simulink model "DeratingControl"  (R2021b)
settings: Solver=VariableStepAuto  StartTime=0.0  StopTime=2  FixedStep=Ts  RelTol=1e-3
model workspace (MAT data in the model file):
  df = Simulink.Parameter
  df.Value = 0.9
  df.DataType = 'auto'
  df.Complexity = 'real'
  df.Dimensions = [1 1]
undefined symbols (not defined in the file): const_facInvTempDera, const_facMotTempDera, const_facPwrDera, const_stDera, const_tiTaskFast, const_tqBattDeraGenLim, const_tqBattDeraMotLim, const_tqDeraGen, const_tqDeraMot, const_tqEmMaxNp1, const_tqInvTempDeraMax, const_tqInvTempDeraMin, const_tqMotTempDeraMax, const_tqMotTempDeraMin, const_tqSpLim, const_tqSpLimMax, const_tqSpLimMin, const_tqTqReq
libraries: simulink x3
settings Model: PacingRate=0.350000  Creator=win  LastModifiedBy=win

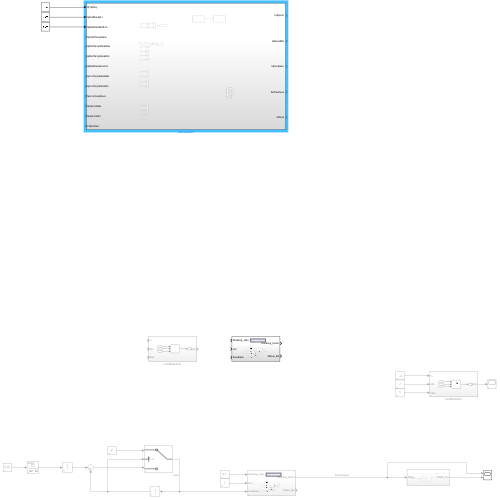
[thumbnail: Simulink's stored preview of the top-level diagram]
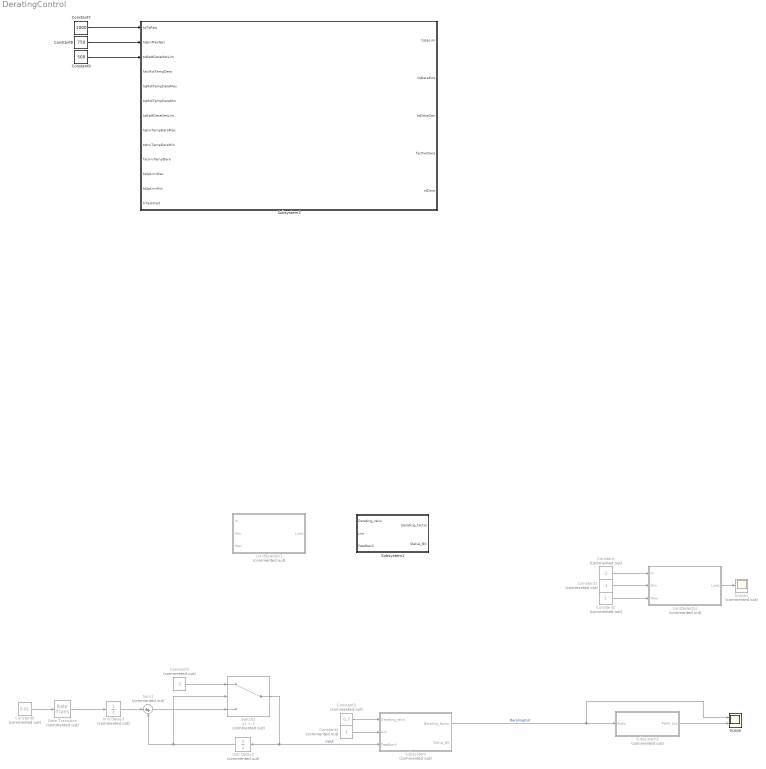
== system DeratingControl ==
  Constant : Constant  Commented=on  Value=-2
  Constant1 : Constant  Commented=on  Value=-1
  Constant2 : Constant  Commented=on
  Constant3 : Constant  Commented=on  Value=-2
  Constant4 : Constant  Commented=on
  Constant5 : Constant  Commented=on  Value=0.7
  Constant6 : Constant  Commented=on  Value=0.01
  Constant7 : Constant  Value=1000  OutDataTypeStr=int32
  Constant8 : Constant  Value=750  OutDataTypeStr=int32
  Constant9 : Constant  Value=500  OutDataTypeStr=int32
  LimitSelector : Subsystem  Commented=on
  LimitSelector1 : Subsystem  Commented=on
  Rate Transition : RateTransition  Commented=on  OutPortSampleTime=1/36000000
  Scope : Scope  NumInputPorts=2
  Scope1 : Scope  Commented=on
  Subsystem : Subsystem  Commented=on
  Subsystem1 : Subsystem
  Subsystem2 : Subsystem  Commented=on
  Subsystem3 : Subsystem  Description=Torque setpoint limit maximum value
  Sum1 : Sum  Commented=on  Inputs=|++
  Switch2 : Switch  Commented=on  Criteria=u2 > Threshold  Threshold=2
  Unit Delay2 : UnitDelay  Commented=on  SampleTime=-1  HasFrameUpgradeWarning=on
  Unit Delay3 : UnitDelay  Commented=on  SampleTime=-1  HasFrameUpgradeWarning=on
  wires:
  Unit Delay2/1 -> Switch2/2, Sum1/2
  Constant3/1 -> Switch2/1
  Sum1/1 -> Switch2/3
  Unit Delay3/1 -> Sum1/1
  Switch2/1 -> Subsystem/3(Feedback), Unit Delay2/1  "input"
  Constant4/1 -> Subsystem/2(Lim)
  Constant5/1 -> Subsystem/1(Derating_ratio)
  Subsystem/1(Derating_factor) -> Scope/1, Subsystem2/1(Ratio)  "DeratingOut"
  Subsystem2/1(PWM_Out) -> Scope/2
  Constant6/1 -> Rate Transition/1
  Rate Transition/1 -> Unit Delay3/1
  Constant/1 -> LimitSelector/1(In)
  Constant1/1 -> LimitSelector/2(Min)
  Constant2/1 -> LimitSelector/3(Max)
  LimitSelector/1(Limit) -> Scope1/1
  Constant7/1 -> Subsystem3/1("tqTqReq ")
  Constant8/1 -> Subsystem3/2("tqEmMaxNp1 ")
  Constant9/1 -> Subsystem3/3(tqBattDeraMotLim)

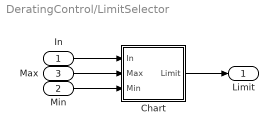
== system DeratingControl/LimitSelector ==
  In : Inport
  Min : Inport  Port=2
  Max : Inport  Port=3
  Chart : Stateflow chart  TreatAsAtomicUnit=on
  Limit : Outport
  wires:
  In/1 -> Chart/1(In)
  Max/1 -> Chart/2(Max)
  Min/1 -> Chart/3(Min)
  Chart/1(Limit) -> Limit/1

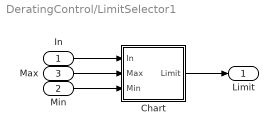
== system DeratingControl/LimitSelector1 ==
  In : Inport
  Min : Inport  Port=2
  Max : Inport  Port=3
  Chart : Stateflow chart  TreatAsAtomicUnit=on
  Limit : Outport
  wires:
  In/1 -> Chart/1(In)
  Max/1 -> Chart/2(Max)
  Min/1 -> Chart/3(Min)
  Chart/1(Limit) -> Limit/1

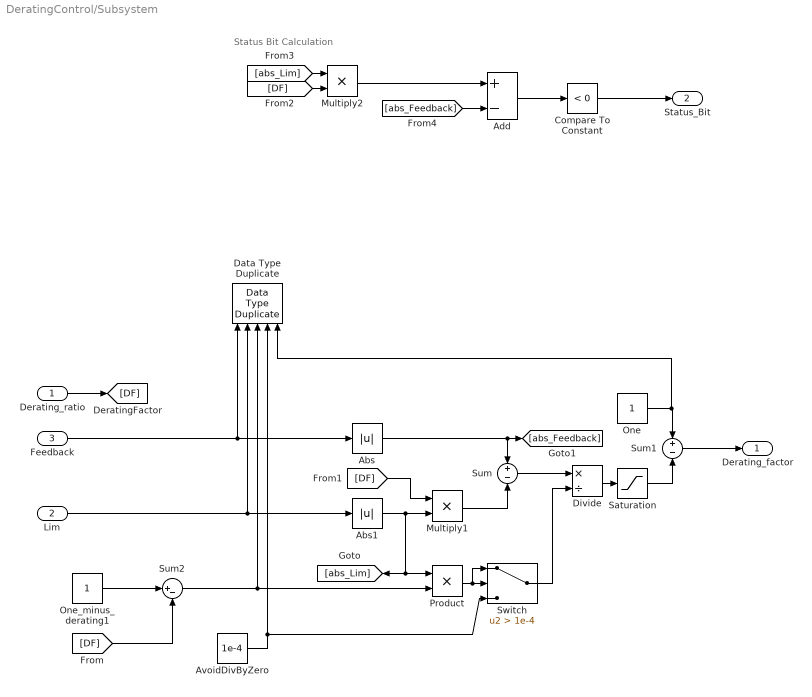
== system DeratingControl/Subsystem ==
  note: Status Bit Calculation
  Derating_ratio : Inport
  Lim : Inport  Port=2
  Feedback : Inport  Port=3
  Abs : Abs  RndMeth=Simplest
  Abs1 : Abs  RndMeth=Simplest
  Add : Sum  Inputs=+-
  AvoidDivByZero : Constant  Value=1e-4  OutDataTypeStr=Inherit: Inherit via back propagation
  Compare To Constant : simulink/Logic and Bit Operations/Compare To Constant  relop=<  const=0  OutDataTypeStr=boolean
  Data Type Duplicate : DataTypeDuplicate  NumInputPorts=5
  Divide : Product  Inputs=*/  RndMeth=Simplest  OutDataTypeStr=Inherit: Same as first input
  Multiply1 : Product  Inputs=**  RndMeth=Simplest  OutDataTypeStr=Inherit: Same as first input
  Multiply2 : Product  Inputs=**  RndMeth=Simplest  OutDataTypeStr=Inherit: Same as first input
  One : Constant  OutDataTypeStr=Inherit: Inherit via back propagation
  One_minus_derating1 : Constant  OutDataTypeStr=Inherit: Inherit via back propagation
  Product : Product  RndMeth=Simplest  OutDataTypeStr=Inherit: Same as first input
  Saturation : Saturate  UpperLimit=1  LowerLimit=0  RndMeth=Simplest
  Sum : Sum  Inputs=+-  RndMeth=Simplest  OutDataTypeStr=Inherit: Same as first input
  Sum1 : Sum  Inputs=+-  RndMeth=Simplest  OutDataTypeStr=Inherit: Same as first input
  Sum2 : Sum  Inputs=|+-
  Switch : Switch  Criteria=u2 > Threshold  Threshold=1e-4
  Derating_factor : Outport  VectorParamsAs1DForOutWhenUnconnected=off
  Status_Bit : Outport  Port=2  OutMin=0  OutMax=1  OutDataTypeStr=boolean  VectorParamsAs1DForOutWhenUnconnected=off
  wires:
  Derating_ratio/1 -> [DF]
  Sum1/1 -> Derating_factor/1
  One/1 -> Sum1/1, Data Type Duplicate/5
  Abs1/1 -> Multiply1/2, Product/1, [abs_Lim]
  Abs/1 -> [abs_Feedback], Sum/1
  Feedback/1 -> Data Type Duplicate/1, Abs/1
  Sum/1 -> Divide/1
  Saturation/1 -> Sum1/2
  Divide/1 -> Saturation/1
  Sum2/1 -> Product/2, Data Type Duplicate/3
  Multiply1/1 -> Sum/2
  Lim/1 -> Abs1/1, Data Type Duplicate/2
  Switch/1 -> Divide/2
  Product/1 -> Switch/1, Switch/2
  AvoidDivByZero/1 -> Data Type Duplicate/4, Switch/3
  [DF] -> Sum2/2
  One_minus_derating1/1 -> Sum2/1
  Add/1 -> Compare To Constant/1
  Compare To Constant/1 -> Status_Bit/1
  [DF] -> Multiply2/2
  Multiply2/1 -> Add/1
  [abs_Lim] -> Multiply2/1
  [abs_Feedback] -> Add/2
  [DF] -> Multiply1/1

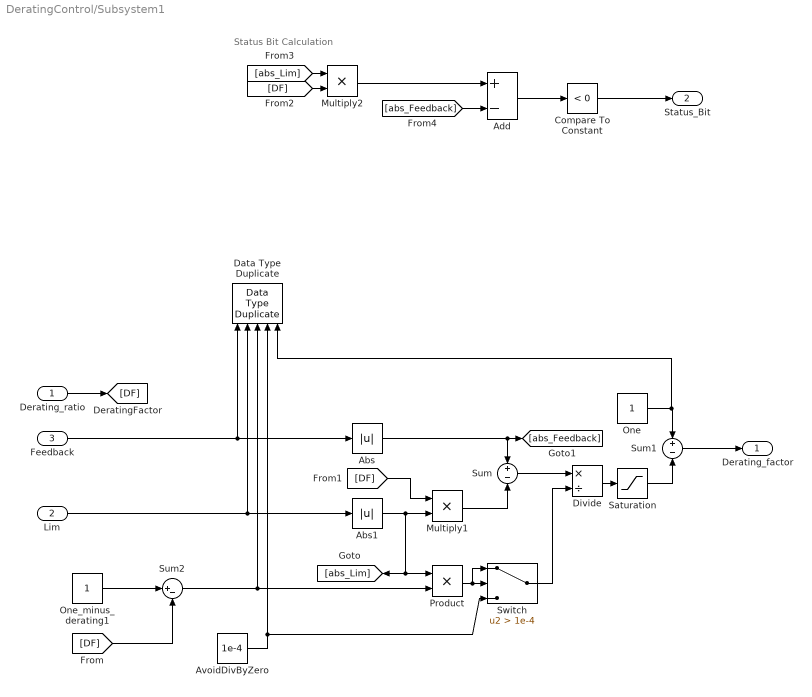
== system DeratingControl/Subsystem1 ==
  note: Status Bit Calculation
  Derating_ratio : Inport
  Lim : Inport  Port=2
  Feedback : Inport  Port=3
  Abs : Abs  RndMeth=Simplest
  Abs1 : Abs  RndMeth=Simplest
  Add : Sum  Inputs=+-
  AvoidDivByZero : Constant  Value=1e-4  OutDataTypeStr=Inherit: Inherit via back propagation
  Compare To Constant : simulink/Logic and Bit Operations/Compare To Constant  relop=<  const=0  OutDataTypeStr=boolean
  Data Type Duplicate : DataTypeDuplicate  NumInputPorts=5
  Divide : Product  Inputs=*/  RndMeth=Simplest  OutDataTypeStr=Inherit: Same as first input
  Multiply1 : Product  Inputs=**  RndMeth=Simplest  OutDataTypeStr=Inherit: Same as first input
  Multiply2 : Product  Inputs=**  RndMeth=Simplest  OutDataTypeStr=Inherit: Same as first input
  One : Constant  OutDataTypeStr=Inherit: Inherit via back propagation
  One_minus_derating1 : Constant  OutDataTypeStr=Inherit: Inherit via back propagation
  Product : Product  RndMeth=Simplest  OutDataTypeStr=Inherit: Same as first input
  Saturation : Saturate  UpperLimit=1  LowerLimit=0  RndMeth=Simplest
  Sum : Sum  Inputs=+-  RndMeth=Simplest  OutDataTypeStr=Inherit: Same as first input
  Sum1 : Sum  Inputs=+-  RndMeth=Simplest  OutDataTypeStr=Inherit: Same as first input
  Sum2 : Sum  Inputs=|+-
  Switch : Switch  Criteria=u2 > Threshold  Threshold=1e-4
  Derating_factor : Outport  VectorParamsAs1DForOutWhenUnconnected=off
  Status_Bit : Outport  Port=2  OutMin=0  OutMax=1  OutDataTypeStr=boolean  VectorParamsAs1DForOutWhenUnconnected=off
  wires:
  [DF] -> Multiply1/1
  [abs_Feedback] -> Add/2
  [abs_Lim] -> Multiply2/1
  Multiply2/1 -> Add/1
  [DF] -> Multiply2/2
  Compare To Constant/1 -> Status_Bit/1
  Add/1 -> Compare To Constant/1
  One_minus_derating1/1 -> Sum2/1
  [DF] -> Sum2/2
  AvoidDivByZero/1 -> Switch/3, Data Type Duplicate/4
  Product/1 -> Switch/2, Switch/1
  Switch/1 -> Divide/2
  Lim/1 -> Data Type Duplicate/2, Abs1/1
  Multiply1/1 -> Sum/2
  Sum2/1 -> Data Type Duplicate/3, Product/2
  Divide/1 -> Saturation/1
  Saturation/1 -> Sum1/2
  Sum/1 -> Divide/1
  Feedback/1 -> Abs/1, Data Type Duplicate/1
  Abs/1 -> Sum/1, [abs_Feedback]
  Abs1/1 -> [abs_Lim], Product/1, Multiply1/2
  One/1 -> Data Type Duplicate/5, Sum1/1
  Sum1/1 -> Derating_factor/1
  Derating_ratio/1 -> [DF]

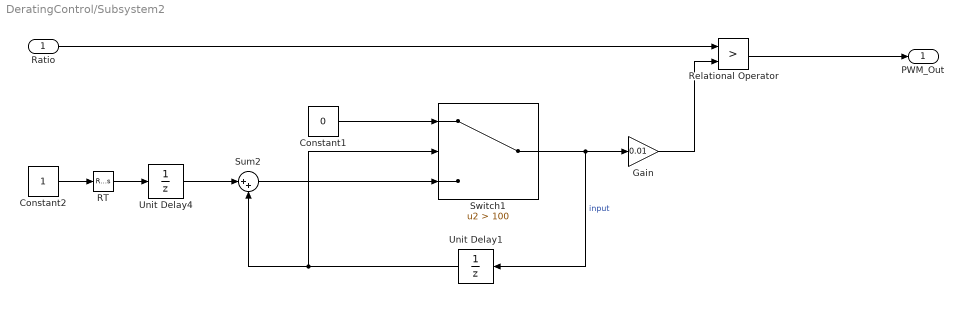
== system DeratingControl/Subsystem2 ==
  Ratio : Inport
  Constant1 : Constant  Value=0
  Constant2 : Constant
  Gain : Gain  Gain=0.01
  RT : RateTransition  Deterministic=off
  Relational Operator : RelationalOperator  Operator=>  OutDataTypeStr=boolean  RndMeth=Simplest
  Sum2 : Sum  Inputs=|++
  Switch1 : Switch  Criteria=u2 > Threshold  Threshold=100
  Unit Delay1 : UnitDelay  SampleTime=-1  HasFrameUpgradeWarning=on
  Unit Delay4 : UnitDelay  SampleTime=-1  HasFrameUpgradeWarning=on
  PWM_Out : Outport
  wires:
  Sum2/1 -> Switch1/3
  Unit Delay1/1 -> Switch1/2, Sum2/2
  Relational Operator/1 -> PWM_Out/1
  Constant2/1 -> RT/1
  Switch1/1 -> Unit Delay1/1, Gain/1  "input"
  Unit Delay4/1 -> Sum2/1
  Ratio/1 -> Relational Operator/1
  RT/1 -> Unit Delay4/1
  Constant1/1 -> Switch1/1
  Gain/1 -> Relational Operator/2

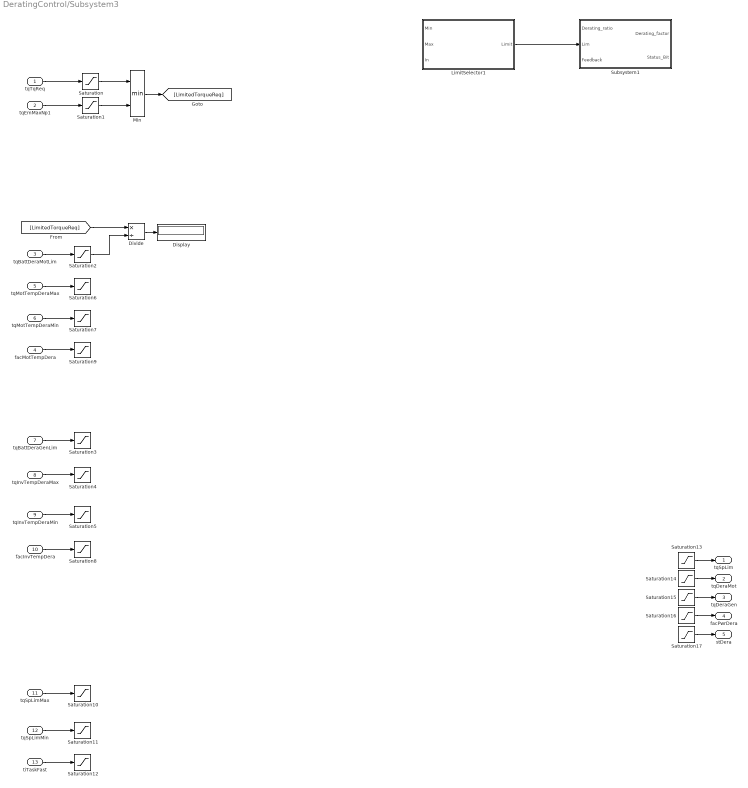
== system DeratingControl/Subsystem3 ==
  "tqTqReq " : Inport  OutMin=const_tqTqReq(1)  OutMax=const_tqTqReq(2)  OutDataTypeStr=int32
  "tqEmMaxNp1 " : Inport  Description=EM Maximum torque N+1 step  Port=2  OutMin=const_tqEmMaxNp1(1)  OutMax=const_tqEmMaxNp1(2)  OutDataTypeStr=int32
  tqBattDeraMotLim : Inport  Description=Derated motor mode torque output according to battery limits  Port=3  OutMin=const_tqBattDeraMotLim(1)  OutMax=const_tqBattDeraMotLim(2)  OutDataTypeStr=int32
  "facMotTempDera " : Inport  Description=Torque derating factor according to motor temperature  Port=4  OutMin=const_facMotTempDera(1)  OutMax=const_facMotTempDera(2)  OutDataTypeStr=int32
  "tqMotTempDeraMax " : Inport  Description=Derated torque maximum value according to motor temperature  Port=5  OutMin=const_tqMotTempDeraMax(1)  OutMax=const_tqMotTempDeraMax(2)  OutDataTypeStr=int32
  "tqMotTempDeraMin " : Inport  Description=Derated torque minimum value according to motor temperature  Port=6  OutMin=const_tqMotTempDeraMin(1)  OutMax=const_tqMotTempDeraMin(2)  OutDataTypeStr=int32
  tqBattDeraGenLim : Inport  Description=Derated generator mode torque output according to battery limits  Port=7  OutMin=const_tqBattDeraGenLim(1)  OutMax=const_tqBattDeraGenLim(2)  OutDataTypeStr=int32
  tqInvTempDeraMax : Inport  Description=Derated torque maximum value according to inverter temperature  Port=8  OutMin=const_tqInvTempDeraMax(1)  OutMax=const_tqInvTempDeraMax(2)  OutDataTypeStr=int32
  tqInvTempDeraMin : Inport  Description=Derated torque minimum value according to inverter temperature  Port=9  OutMin=const_tqInvTempDeraMin(1)  OutMax=const_tqInvTempDeraMin(2)  OutDataTypeStr=int32
  "facInvTempDera " : Inport  Description=Torque derating factor according to inverter temperature  Port=10  OutMin=const_facInvTempDera(1)  OutMax=const_facInvTempDera(2)  OutDataTypeStr=int32
  "tqSpLimMax " : Inport  Port=11  OutMin=const_tqSpLimMax(1)  OutMax=const_tqSpLimMax(2)  OutDataTypeStr=int32
  "tqSpLimMin " : Inport  Description=Torque setpoint limit minimum value  Port=12  OutMin=const_tqSpLimMin(1)  OutMax=const_tqSpLimMin(2)  OutDataTypeStr=int32
  "tiTaskFast " : Inport  Description=Time for the fast task (PWM task)  Port=13  OutMin=const_tiTaskFast(1)  OutMax=const_tiTaskFast(2)  OutDataTypeStr=int32
  Display : Display
  Divide : Product  Inputs=*/  OutMin=0  OutMax=1  OutDataTypeStr=int32
  LimitSelector1 : Subsystem
  Min : MinMax  Inputs=2
  Saturation : Saturate  UpperLimit=const_tqTqReq(2)  LowerLimit=const_tqTqReq(1)
  Saturation1 : Saturate  UpperLimit=const_tqEmMaxNp1(2)  LowerLimit=const_tqEmMaxNp1(1)
  Saturation10 : Saturate  UpperLimit=const_tqSpLimMax(2)  LowerLimit=const_tqSpLimMax(1)  OutDataTypeStr=int32
  Saturation11 : Saturate  UpperLimit=const_tqSpLimMin(2)  LowerLimit=const_tqSpLimMin(1)  OutDataTypeStr=int32
  Saturation12 : Saturate  UpperLimit=const_tiTaskFast(2)  LowerLimit=const_tiTaskFast(1)  OutDataTypeStr=int32
  Saturation13 : Saturate  UpperLimit=const_tqSpLim(2)  LowerLimit=const_tqSpLim(1)
  Saturation14 : Saturate  UpperLimit=const_tqDeraMot(2)  LowerLimit=const_tqDeraMot(1)
  Saturation15 : Saturate  UpperLimit=const_tqDeraGen(2)  LowerLimit=const_tqDeraGen(1)
  Saturation16 : Saturate  UpperLimit=const_facPwrDera(2)  LowerLimit=const_facPwrDera(1)
  Saturation17 : Saturate  UpperLimit=const_stDera(2)  LowerLimit=const_stDera(1)
  Saturation2 : Saturate  UpperLimit=const_tqBattDeraMotLim(2)  LowerLimit=const_tqBattDeraMotLim(1)
  Saturation3 : Saturate  UpperLimit=const_tqBattDeraGenLim(2)  LowerLimit=const_tqBattDeraGenLim(1)
  Saturation4 : Saturate  UpperLimit=const_tqInvTempDeraMax(2)  LowerLimit=const_tqInvTempDeraMax(1)  OutDataTypeStr=int32
  Saturation5 : Saturate  UpperLimit=const_tqInvTempDeraMin(2)  LowerLimit=const_tqInvTempDeraMin(1)  OutDataTypeStr=int32
  Saturation6 : Saturate  UpperLimit=const_tqMotTempDeraMax(2)  LowerLimit=const_tqMotTempDeraMax(1)  OutDataTypeStr=int32
  Saturation7 : Saturate  UpperLimit=const_tqMotTempDeraMin(2)  LowerLimit=const_tqMotTempDeraMin(1)  OutDataTypeStr=int32
  Saturation8 : Saturate  UpperLimit=const_facInvTempDera(2)  LowerLimit=const_facInvTempDera(1)  OutDataTypeStr=int32
  Saturation9 : Saturate  UpperLimit=const_facMotTempDera(2)  LowerLimit=const_facMotTempDera(1)  OutDataTypeStr=int32
  Subsystem1 : Subsystem
  "tqSpLim " : Outport  Description=Limited torque setpoint  OutMin=const_tqSpLim(1)  OutMax=const_tqSpLim(2)
  "tqDeraMot " : Outport  Description=Derated torque for motor mode  Port=2  OutMin=const_tqDeraMot(1)  OutMax=const_tqDeraMot(2)
  "tqDeraGen " : Outport  Description=Derated torque for generator mode  Port=3  OutMin=const_tqDeraGen(1)  OutMax=const_tqDeraGen(2)
  "facPwrDera " : Outport  Description=Power derating factor  Port=4  OutMin=const_facPwrDera(1)  OutMax=const_facPwrDera(2)
  "stDera " : Outport  Description=Derating status  Port=5  OutMin=const_stDera(1)  OutMax=const_stDera(2)
  wires:
  "tqTqReq "/1 -> Saturation/1
  "tqEmMaxNp1 "/1 -> Saturation1/1
  tqBattDeraMotLim/1 -> Saturation2/1
  tqBattDeraGenLim/1 -> Saturation3/1
  tqInvTempDeraMax/1 -> Saturation4/1
  tqInvTempDeraMin/1 -> Saturation5/1
  "tqMotTempDeraMax "/1 -> Saturation6/1
  "tqMotTempDeraMin "/1 -> Saturation7/1
  "facInvTempDera "/1 -> Saturation8/1
  "tqSpLimMax "/1 -> Saturation10/1
  "facMotTempDera "/1 -> Saturation9/1
  "tqSpLimMin "/1 -> Saturation11/1
  "tiTaskFast "/1 -> Saturation12/1
  Saturation13/1 -> "tqSpLim "/1
  Saturation14/1 -> "tqDeraMot "/1
  Saturation15/1 -> "tqDeraGen "/1
  Saturation16/1 -> "facPwrDera "/1
  Saturation17/1 -> "stDera "/1
  LimitSelector1/1(Limit) -> Subsystem1/2(Lim)
  Saturation/1 -> Min/1
  Saturation1/1 -> Min/2
  Min/1 -> [LimitedTorqueReq]
  Divide/1 -> Display/1
  Saturation2/1 -> Divide/2
  [LimitedTorqueReq] -> Divide/1

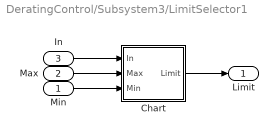
== system DeratingControl/Subsystem3/LimitSelector1 ==
  Min : Inport
  Max : Inport  Port=2
  In : Inport  Port=3
  Chart : Stateflow chart  TreatAsAtomicUnit=on
  Limit : Outport
  wires:
  In/1 -> Chart/1(In)
  Max/1 -> Chart/2(Max)
  Min/1 -> Chart/3(Min)
  Chart/1(Limit) -> Limit/1

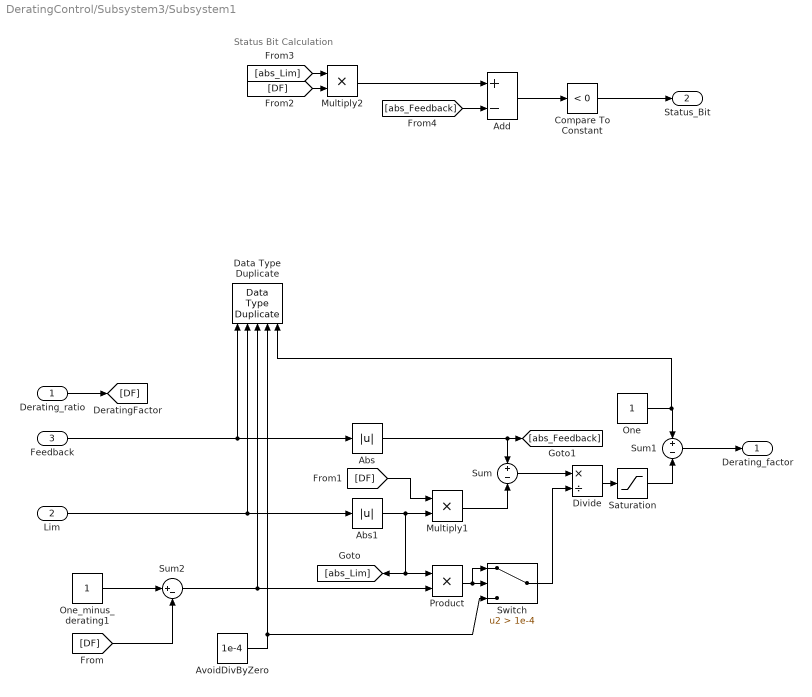
== system DeratingControl/Subsystem3/Subsystem1 ==
  note: Status Bit Calculation
  Derating_ratio : Inport
  Lim : Inport  Port=2
  Feedback : Inport  Port=3
  Abs : Abs  RndMeth=Simplest
  Abs1 : Abs  RndMeth=Simplest
  Add : Sum  Inputs=+-
  AvoidDivByZero : Constant  Value=1e-4  OutDataTypeStr=Inherit: Inherit via back propagation
  Compare To Constant : simulink/Logic and Bit Operations/Compare To Constant  relop=<  const=0  OutDataTypeStr=boolean
  Data Type Duplicate : DataTypeDuplicate  NumInputPorts=5
  Divide : Product  Inputs=*/  RndMeth=Simplest  OutDataTypeStr=Inherit: Same as first input
  Multiply1 : Product  Inputs=**  RndMeth=Simplest  OutDataTypeStr=Inherit: Same as first input
  Multiply2 : Product  Inputs=**  RndMeth=Simplest  OutDataTypeStr=Inherit: Same as first input
  One : Constant  OutDataTypeStr=Inherit: Inherit via back propagation
  One_minus_derating1 : Constant  OutDataTypeStr=Inherit: Inherit via back propagation
  Product : Product  RndMeth=Simplest  OutDataTypeStr=Inherit: Same as first input
  Saturation : Saturate  UpperLimit=1  LowerLimit=0  RndMeth=Simplest
  Sum : Sum  Inputs=+-  RndMeth=Simplest  OutDataTypeStr=Inherit: Same as first input
  Sum1 : Sum  Inputs=+-  RndMeth=Simplest  OutDataTypeStr=Inherit: Same as first input
  Sum2 : Sum  Inputs=|+-
  Switch : Switch  Criteria=u2 > Threshold  Threshold=1e-4
  Derating_factor : Outport  VectorParamsAs1DForOutWhenUnconnected=off
  Status_Bit : Outport  Port=2  OutMin=0  OutMax=1  OutDataTypeStr=boolean  VectorParamsAs1DForOutWhenUnconnected=off
  wires:
  [DF] -> Multiply1/1
  [abs_Feedback] -> Add/2
  [abs_Lim] -> Multiply2/1
  Multiply2/1 -> Add/1
  [DF] -> Multiply2/2
  Compare To Constant/1 -> Status_Bit/1
  Add/1 -> Compare To Constant/1
  One_minus_derating1/1 -> Sum2/1
  [DF] -> Sum2/2
  AvoidDivByZero/1 -> Switch/3, Data Type Duplicate/4
  Product/1 -> Switch/2, Switch/1
  Switch/1 -> Divide/2
  Lim/1 -> Data Type Duplicate/2, Abs1/1
  Multiply1/1 -> Sum/2
  Sum2/1 -> Data Type Duplicate/3, Product/2
  Divide/1 -> Saturation/1
  Saturation/1 -> Sum1/2
  Sum/1 -> Divide/1
  Feedback/1 -> Abs/1, Data Type Duplicate/1
  Abs/1 -> Sum/1, [abs_Feedback]
  Abs1/1 -> [abs_Lim], Product/1, Multiply1/2
  One/1 -> Data Type Duplicate/5, Sum1/1
  Sum1/1 -> Derating_factor/1
  Derating_ratio/1 -> [DF]

== stateflow chart DeratingControl/LimitSelector1/Chart ==
  state LimitSelector
    Limit= Max;
  state Min
    Limit=Min;
  (default) -> LimitSelector
  LimitSelector -> Min : [In < Min]
  Min -> LimitSelector : [[In >= Min]]
  data: In input; Max input; Min input; Limit output

== stateflow chart DeratingControl/Subsystem3/LimitSelector1/Chart ==
  state LimitSelector
    Limit= Max;
  state Min
    Limit=Min;
  (default) -> LimitSelector
  LimitSelector -> Min : [In < Min]
  Min -> LimitSelector : [[In >= Min]]
  data: In input; Max input; Min input; Limit output

== stateflow chart DeratingControl/LimitSelector/Chart ==
  state LimitSelector
    Limit= Max;
  state Min
    Limit=Min;
  (default) -> LimitSelector
  LimitSelector -> Min : [In < Min]
  Min -> LimitSelector : [[In >= Min]]
  data: In input; Max input; Min input; Limit output
